simulink subsystem "EISFirmware"  (R2022a)
settings: Solver=VariableStepAuto  StartTime=0.0  StopTime=10.0  RelTol=1e-3
undefined symbols (not defined in the file): Call, Function
settings Model: Creator=mateu  LastModifiedBy=mateu

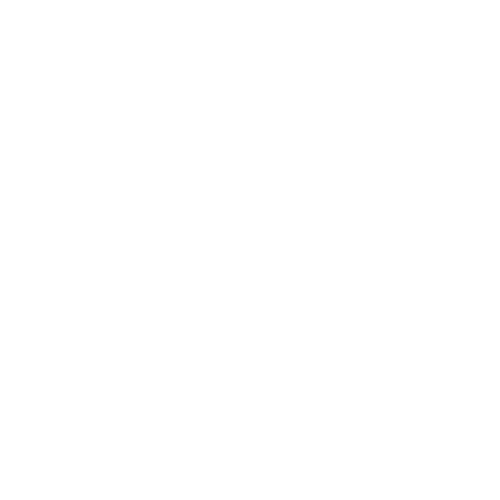
[thumbnail: Simulink's stored preview of the top-level diagram]
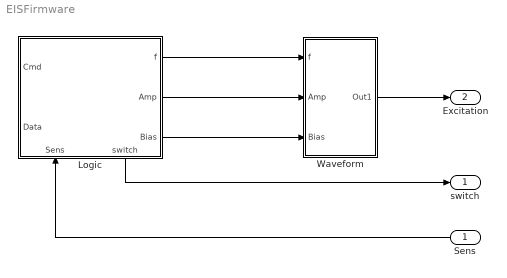
== system EISFirmware ==
  Sens : Inport
  Logic : Subsystem
      settings: PortSchema="{\"entries\":[{\"content\":{\"sides\":[{\"content\":{\"connectorIds\":[\"In1\",\"Out5\"]},\"type\":\"ConnectorPlacement.EquallySpacedRectSide\",\"uuid\":\"d56ad198-652c-4256-842a-109e5accf008\"},{\"content\":{\"connectorIds\":[\"Out1\",\"Out2\",\"Out3\"],\"side\":\"RIGHT\"},\"type\":\"ConnectorPlacement.EquallySpacedRectSide\",\"uuid\":\"47c51815-899b-4ad2-8de7-b4874420b12f\"},{\"content\":{\"connectorIds\":[],\"side\":\"TOP\"},\"type\":\"ConnectorPlacement.EquallySpacedRectSide\",\"uuid\":\"c9d07e47-4fb4-4668-93cc-5b7350b95114\"},{\"content\":{\"connectorIds\":[\"In2\",\"Out4\"],\"side\":\"BOTTOM\"},\"type\":\"ConnectorPlacement.EquallySpacedRectSide\",\"uuid\":\"c58de459-fdb1-4cb8-a48b-116fc9204598\"}]},\"type\":\"ConnectorPlacement.EquallySpacedConnector\",\"uuid\":\"68e0456f-f712-40c9-b6ff-129aa0b1f4b6\"}],\"packageUris\":[\"http://schema.mathworks.com/mf0/Connector/R2020b\"],\"version\":\"1.0\"}"
  Waveform : Subsystem
  switch : Outport
  Excitation : Outport  Port=2
  wires:
  Waveform/1(Out1) -> Excitation/1
  Logic/1(f) -> Waveform/1(f)
  Logic/2(Amp) -> Waveform/2(Amp)
  Logic/3(Bias) -> Waveform/3(Bias)
  Logic/4(switch) -> switch/1
  Sens/1 -> Logic/2(Sens)

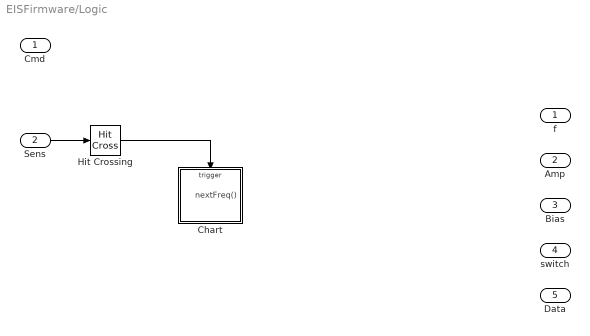
== system EISFirmware/Logic ==
  Cmd : Inport
  Sens : Inport  Port=2
  Chart : Stateflow chart  TreatAsAtomicUnit=on
  Hit Crossing : HitCross  HitCrossingDirection=rising  HitCrossingOutputType=Function-Call
  f : Outport
  Amp : Outport  Port=2
  Bias : Outport  Port=3
  switch : Outport  Port=4
  Data : Outport  Port=5
  wires:
  Hit Crossing/1 -> Chart/Trigger
  Sens/1 -> Hit Crossing/1

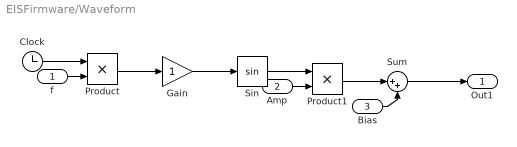
== system EISFirmware/Waveform ==
  f : Inport
  Amp : Inport  Port=2
  Bias : Inport  Port=3
  Clock : Clock
  Gain : Gain
  Product : Product
  Product1 : Product
  Sin : Trigonometry
  Sum : Sum  Inputs=|++
  Out1 : Outport
  wires:
  Sum/1 -> Out1/1
  Product1/1 -> Sum/1
  Bias/1 -> Sum/2
  f/1 -> Product/2
  Product/1 -> Gain/1
  Gain/1 -> Sin/1
  Clock/1 -> Product/1
  Sin/1 -> Product1/1
  Amp/1 -> Product1/2

== stateflow chart EISFirmware/Logic/Chart ==
  state Idle
  state NextFreq
  NextFreq -> Idle
  (default) -> Idle
  Idle -> NextFreq : after(5,T){send(nextFreq)}
  events: T input FUNCTION_CALL_EVENT; nextFreq output FUNCTION_CALL_EVENT
